simulink model "vehicle"  (R2016b)
settings: Solver=ode4  StartTime=0.0  StopTime=Inf  FixedStep=0.003  RelTol=1e-3
settings Model: Creator=ANTO_  LastModifiedBy=ANTO_
settings DebuggingCC: RootOutportRequireBusObject=error  StrictBusMsg=ErrorOnBusTreatedAsVector
settings HardwareCC: ProdBitPerPointer=32  ProdBitPerSizeT=32  ProdBitPerPtrDiffT=32  ProdLargestAtomicInteger=Long  ProdWordSize=32  ProdHWDeviceType=ARM Compatible->ARM 7
settings RTWCC: SystemTargetFile=NIVeriStand_Linux_ARM_32.tlc  TemplateMakefile=NIVeriStand_Linux_ARM_32.tmf  Description=NI Linux Real-Time ARM (32-bit) Target
settings STFCustomTargetCC: TargetLangStandard=C99 (ISO)  MatFileLogging=on  MATLABClassNameForMDSCustomization=Simulink.SoftwareTarget.TargetSpecificTriggerConfigurationBase  SystemTargetFile=NIVeriStand_Linux_ARM_32.tlc

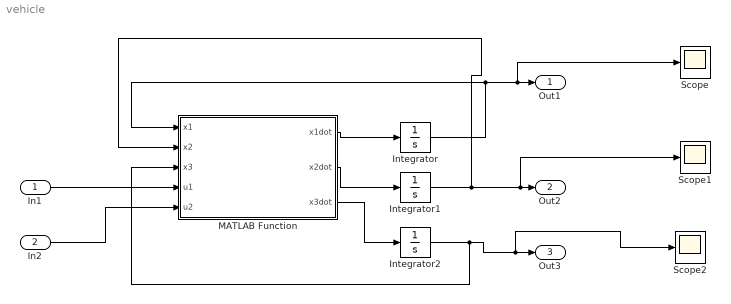
== system vehicle ==
  In1 : Inport
  In2 : Inport  Port=2
  Integrator : Integrator  InitialCondition=0.6
  Integrator1 : Integrator  InitialCondition=0.6
  Integrator2 : Integrator
  MATLAB Function : MATLAB Function  TreatAsAtomicUnit=on
  Scope : Scope
  Scope1 : Scope
  Scope2 : Scope
  Out1 : Outport
  Out2 : Outport  Port=2
  Out3 : Outport  Port=3
  wires:
  MATLAB Function/1(x1dot) -> Integrator/1
  MATLAB Function/2(x2dot) -> Integrator1/1
  Integrator/1 -> MATLAB Function/1(x1), Scope/1, Out1/1
  Integrator1/1 -> Scope1/1, Out2/1, MATLAB Function/2(x2)
  In1/1 -> MATLAB Function/4(u1)
  In2/1 -> MATLAB Function/5(u2)
  MATLAB Function/3(x3dot) -> Integrator2/1
  Integrator2/1 -> MATLAB Function/3(x3), Scope2/1, Out3/1

== matlab function vehicle/MATLAB Function ==
  data: x1 input; x2 input; x3 input; x1dot output; x2dot output; u1 input; u2 input; x3dot output
function [x1dot,x2dot,x3dot] = Boost_DC_converter(x1,x2,x3,u1,u2)

  x = [x1;x2;x3];
  
  dxdt = zeros(3,1);
  c=atan(tan(u2)/2);

  dxdt(1)=u1*cos(c+x(3))/cos(c);
  dxdt(2)=u1*sin(c+x(3))/cos(c);
  dxdt(3)=u1*tan(u2);
  
  x1dot = dxdt(1);
  x2dot = dxdt(2);
  x3dot = dxdt(3);

end
